simulink model "Daolibai_design_OSFtu"  (R2016a)
settings: Solver=VariableStepAuto  SolverMode=SingleTasking  StartTime=0.0  StopTime=10.0  RelTol=1e-3
values from neighbouring files (symbols this model uses):
  A = [-18/7 9 0;1 -1 1;0 -14.28 0]    [Caishidianlu_design.m]    (also in Daolibai_analysis_ControllAndObserv.m = [0 1 0 0; Daolibai_analysis_stability.m = [0 1 0 0; Daolibai_design_OSF.m = [0 1 0 0; Daolibai_design_OSFandPIOF.m = [0 1 0 0)
  A1 = [0 1 0 0 ... (first row only)    [Daolibai_analysis_ControllAndObserv.m]    (also in Daolibai_analysis_stability.m; Daolibai_design_OSF.m; Daolibai_design_OSFandPIOF.m = [A [0 0 0 0]'; Daolibai_design_SF.m)
  B = [27/7;0;0]    [Caishidianlu_design.m]    (also in Daolibai_analysis_ControllAndObserv.m = [0;1;0;-2]; Daolibai_analysis_stability.m = [0;1;0;-2]; Daolibai_design_OSF.m = [0;1;0;-2]; Daolibai_design_OSFandPIOF.m = [0;1;0;-2])
  B1 = [0;1;0;-2]    [Daolibai_analysis_ControllAndObserv.m]    (also in Daolibai_analysis_stability.m; Daolibai_design_OSF.m; Daolibai_design_OSFandPIOF.m = [B;0]; Daolibai_design_SF.m)
  C = [1 0 0]    [Caishidianlu_design.m]    (also in Daolibai_analysis_ControllAndObserv.m = [1 0 0 0]; Daolibai_analysis_stability.m = [1 0 0 0]; Daolibai_design_OSF.m = [1 0 0 0]; Daolibai_design_OSFandPIOF.m = [1 0 0 0])
  C1 = [1 0 0 0]    [Daolibai_analysis_ControllAndObserv.m]    (also in Daolibai_analysis_stability.m; Daolibai_design_OSF.m; Daolibai_design_SF.m; Daolibai_design_SFandOF.m)
  D = [1 0 0]    [Caishidianlu_design.m]    (also in Daolibai_analysis_ControllAndObserv.m = [0]; Daolibai_analysis_stability.m = [0]; Daolibai_design_OSF.m = [0]; Daolibai_design_OSFandPIOF.m = [0])
  G = G'    [Daolibai_design_OSF.m]    (also in Daolibai_design_OSFandPIOF.m)
  Init = [0.1 0.1 0.5 0.5]    [Daolibai_design_OSF.m]    (also in Daolibai_design_OSFandPIOF.m = [0 0.04 0.005 0.1 ]; Daolibai_design_SFandOF.m; Daolibai_design_SFandPIOF.m = [0 0.1 0.005 0.1 ])
  Initobserv = [0.1 0.1 0.4 0.3]    [Daolibai_design_OSF.m]    (also in Daolibai_design_OSFandPIOF.m = [0 0.015 0 0.1])
  K = inv(P1)*V1    [Caishidianlu_design.m]    (also in Daolibai_design_OSF.m = acker(A1,B1,P1); Daolibai_design_OSFandPIOF.m = acker(A1,B1,P); Daolibai_design_SF.m = acker(A1,B1,P); Daolibai_design_SFandOF.m = acker(A,B,P))
settings Model: Creator=19017  LastModifiedBy=19017
settings DataIOCC: ReturnWorkspaceOutputs=on
settings DebuggingCC: SFUnexpectedBacktrackingDiag=error  SFNoUnconditionalDefaultTransitionDiag=error
settings SFSimCC: SimUseLocalCustomCode=on
settings RTWCC: RTWUseLocalCustomCode=on
settings GRTTargetCC: TargetLangStandard=C99 (ISO)
settings ConfigComp: CovMetricSettings=dwe  CovSaveCumulativeToWorkspaceVar=off  CovSaveSingleToWorkspaceVar=off  CovExternalEMLEnable=on

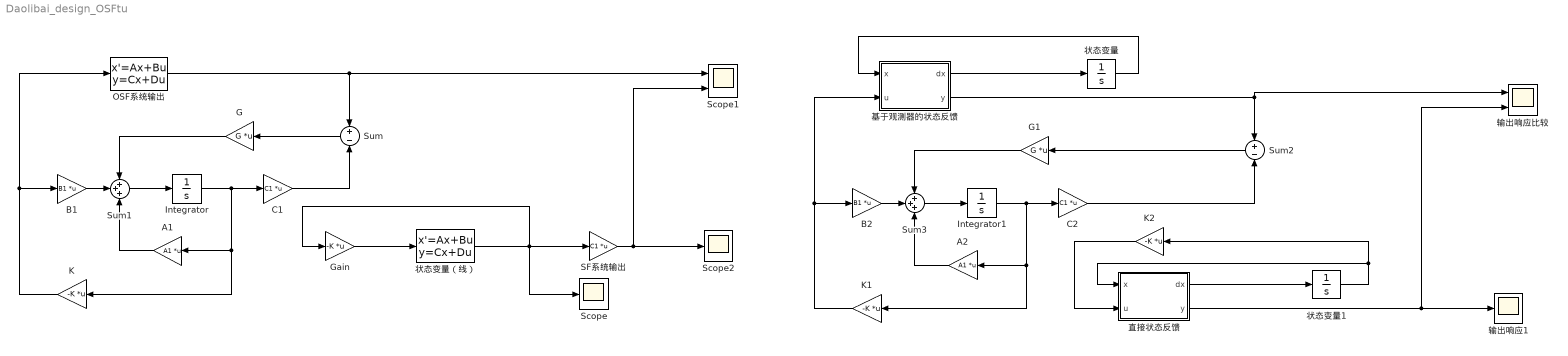
== system Daolibai_design_OSFtu ==
  A1 : Gain  Gain=A1  Multiplication=Matrix(K*u)
  A2 : Gain  Gain=A1  Multiplication=Matrix(K*u)
  B1 : Gain  Gain=B1  Multiplication=Matrix(K*u)
  B2 : Gain  Gain=B1  Multiplication=Matrix(K*u)
  C1 : Gain  Gain=C1  Multiplication=Matrix(K*u)
  C2 : Gain  Gain=C1  Multiplication=Matrix(K*u)
  G : Gain  Gain=G  Multiplication=Matrix(K*u)
  G1 : Gain  Gain=G  Multiplication=Matrix(K*u)
  Gain : Gain  Gain=-K  Multiplication=Matrix(K*u)
  Integrator : Integrator  InitialCondition=Initobserv
  Integrator1 : Integrator  InitialCondition=Initobserv
  K : Gain  Gain=-K  Multiplication=Matrix(K*u)
  K1 : Gain  Gain=-K  Multiplication=Matrix(K*u)
  K2 : Gain  Gain=-K  Multiplication=Matrix(K*u)
  OSF系统输出 : StateSpace  A=A  B=B  C=C  D=D  X0=Init
  SF系统输出 : Gain  Gain=C1  Multiplication=Matrix(K*u)
  Scope : Scope
  Scope1 : Scope  NumInputPorts=2
  Scope2 : Scope
  Sum : Sum  Inputs=+|-
  Sum1 : Sum  Inputs=+++
  Sum2 : Sum  Inputs=+|-
  Sum3 : Sum  Inputs=+++
  基于观测器的状态反馈 : MATLAB Function  TreatAsAtomicUnit=on
  状态变量 : Integrator  InitialCondition=Init
  状态变量1 : Integrator  InitialCondition=Init
  状态变量（线） : StateSpace  A=A  B=B  C=eye(4)  D=[0;0;0;0]  X0=Init
  直接状态反馈 : MATLAB Function  TreatAsAtomicUnit=on
  输出响应1 : Scope
  输出响应比较 : Scope  NumInputPorts=2
  wires:
  OSF系统输出/1 -> Sum/1, Scope1/1
  C1/1 -> Sum/2
  Sum/1 -> G/1
  G/1 -> Sum1/1
  B1/1 -> Sum1/2
  Sum1/1 -> Integrator/1
  A1/1 -> Sum1/3
  Integrator/1 -> A1/1, K/1, C1/1
  SF系统输出/1 -> Scope1/2, Scope2/1
  Gain/1 -> 状态变量（线）/1
  状态变量（线）/1 -> Gain/1, SF系统输出/1, Scope/1
  K/1 -> OSF系统输出/1, B1/1
  C2/1 -> Sum2/2
  B2/1 -> Sum3/2
  Sum2/1 -> G1/1
  Integrator1/1 -> A2/1, K1/1, C2/1
  A2/1 -> Sum3/3
  Sum3/1 -> Integrator1/1
  G1/1 -> Sum3/1
  K1/1 -> 基于观测器的状态反馈/2(u), B2/1
  基于观测器的状态反馈/1(dx) -> 状态变量/1
  状态变量/1 -> 基于观测器的状态反馈/1(x)
  基于观测器的状态反馈/2(y) -> 输出响应比较/1, Sum2/1
  状态变量1/1 -> K2/1, 直接状态反馈/1(x)
  直接状态反馈/1(dx) -> 状态变量1/1
  直接状态反馈/2(y) -> 输出响应比较/2, 输出响应1/1
  K2/1 -> 直接状态反馈/2(u)

== matlab function Daolibai_design_OSFtu/基于观测器的状态反馈 ==
  data: dx output; x input; u input; y output
function [dx,y] = fcn(x,u)
M = 1;
m = 0.1;
l = 0.5;
g = 9.8;
x1=x(1);
x2=x(2);
x3=x(3);
x4=x(4);
dx1 = x2;
dx2 =(u + m*l*x4*x4*sin(x3) - m*g*sin(x3)*cos(x3))/(M + m - m*cos(x3)*cos(x3));
dx3 = x4;
dx4 =(-u*cos(x3) + (M+m)*g*sin(x3) - m*l*x4*x4*sin(x3)*cos(x3))/((M+m)*l - m*l*cos(x3)*cos(x3));
dx = [dx1;dx2;dx3;dx4];
y = x1;

== matlab function Daolibai_design_OSFtu/直接状态反馈 ==
  data: dx output; x input; u input; y output
function [dx,y] = fcn(x,u)
M = 1;
m = 0.1;
l = 0.5;
g = 9.8;
x1=x(1);
x2=x(2);
x3=x(3);
x4=x(4);
dx1 = x2;
dx2 =(u + m*l*x4*x4*sin(x3) - m*g*sin(x3)*cos(x3))/(M + m - m*cos(x3)*cos(x3));
dx3 = x4;
dx4 =(-u*cos(x3) + (M+m)*g*sin(x3) - m*l*x4*x4*sin(x3)*cos(x3))/((M+m)*l - m*l*cos(x3)*cos(x3));
dx = [dx1;dx2;dx3;dx4];
y = x1;
